simulink model "FK_IK"  (R2022b)
settings: Solver=FixedStepAuto  StartTime=0.0  StopTime=10.0  FixedStep=0.01  RelTol=1e-3
settings Model: Creator=Admin  LastModifiedBy=Admin

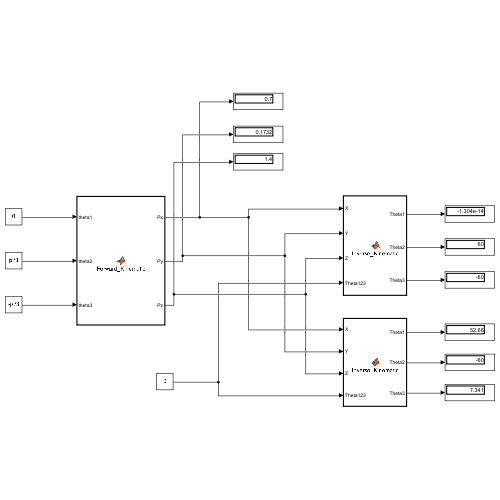
[thumbnail: Simulink's stored preview of the top-level diagram]
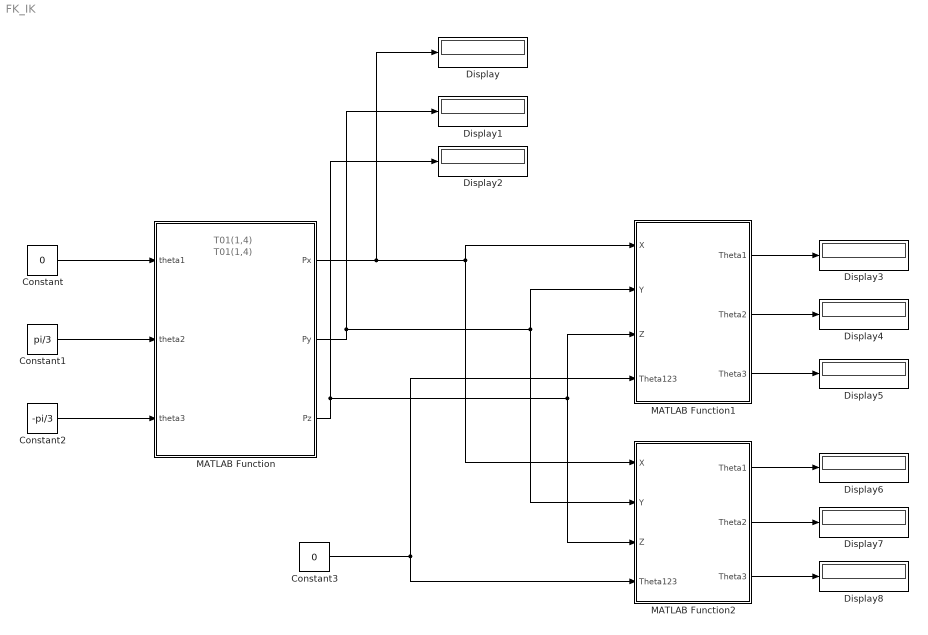
== system FK_IK ==
  note: T01(1,4)
  note: T01(1,4)
  Constant : Constant  Value=0
  Constant1 : Constant  Value=pi/3
  Constant2 : Constant  Value=-pi/3
  Constant3 : Constant  Value=0
  Display{,1..8} (9 alike) : Display
  MATLAB Function : MATLAB Function  TreatAsAtomicUnit=on
  MATLAB Function1 : MATLAB Function  TreatAsAtomicUnit=on
  MATLAB Function2 : MATLAB Function  TreatAsAtomicUnit=on
  wires:
  Constant/1 -> MATLAB Function/1(theta1)
  Constant1/1 -> MATLAB Function/2(theta2)
  Constant2/1 -> MATLAB Function/3(theta3)
  MATLAB Function/1(Px) -> MATLAB Function2/1(X), MATLAB Function1/1(X), Display/1
  MATLAB Function/2(Py) -> MATLAB Function2/2(Y), MATLAB Function1/2(Y), Display1/1
  MATLAB Function/3(Pz) -> MATLAB Function2/3(Z), MATLAB Function1/3(Z), Display2/1
  Constant3/1 -> MATLAB Function2/4(Theta123), MATLAB Function1/4(Theta123)
  MATLAB Function1/1(Theta1) -> Display3/1
  MATLAB Function1/2(Theta2) -> Display4/1
  MATLAB Function1/3(Theta3) -> Display5/1
  MATLAB Function2/3(Theta3) -> Display8/1
  MATLAB Function2/2(Theta2) -> Display7/1
  MATLAB Function2/1(Theta1) -> Display6/1

== matlab function FK_IK/MATLAB Function1 ==
  data: X input; Theta1 output; Y input; Z input; Theta123 input; Theta2 output; Theta3 output
function [Theta1,Theta2,Theta3] = Inverse_Kinematic(X,Y,Z, Theta123)
L0=0.2; L1=0.2; L2=0.25; L3=0.2; L4=0.15;
%% Tinh theta 2
N = X - L1 - L4*cosd(Theta123);
M = Y - L4*sind(Theta123);
C_T2 = (N^2 + M^2 - L2^2 - L3^2) / (2*L2*L3);
S_T2 = sqrt(abs(1 - C_T2^2));
Theta2 = atan2d(S_T2,C_T2);

%% Tinh theta 1
C_T1 = (N*(L2+L3*cosd(Theta2)) + M*L3*sind(Theta2)) / (L2^2+2*L2*L3*cosd(Theta2)+L3^2);
S_T1 = (M*(L2+L3*cosd(Theta2)) - N*L3*sind(Theta2)) / (L2^2+2*L2*L3*cosd(Theta2)+L3^2);
Theta1 = atan2d(S_T1,C_T1);

%% Tinh theta 3
Theta3 = Theta123 - Theta1 - Theta2;

== matlab function FK_IK/MATLAB Function ==
  data: theta1 input; Px output; theta2 input; theta3 input; Py output; Pz output
function [Px,Py,Pz] = Forward_Kinematic(theta1,theta2,theta3)
d1 = 0.3; d2 = 0.3; d3 = 0.3; d4 = 0.3;
L0=0.2; L1=0.2; L2=0.25; L3=0.2; L4=0.15;

%% The individual transformation:
%Ma tran chuyen doi tu he 0 sang 1
T01 = [cos(theta1), -sin(theta1), 0, L1;
       sin(theta1),  cos(theta1), 0,  0;
                  0,             0, 1, L0 + d1 + d2;
                  0,             0, 0,  1];
%Ma tran chuyen doi tu he 1 sang 2
T12 = [cos(theta2), -sin(theta2), 0, L2;
       sin(theta2),  cos(theta2), 0,  0;
                  0,             0, 1,  d3;
                  0,             0, 0,  1];
%Ma tran chuyen doi tu he 2 sang 3
T23 = [cos(theta3), -sin(theta3), 0, L3;
       sin(theta3),  cos(theta3), 0,  0;
                  0,             0, 1,  d4;
                  0,             0, 0,  1];
%Ma tran chuyen doi tu he 2 sang 3
T34 = [1, 0, 0, L4
       0, 1, 0,  0
       0, 0, 1,  0
       0, 0, 0,  1];
% %% The transformation matrix between frame(0) and frame (3)
T04=T01*T12*T23*T34;
%% Position of end-effector
Px = T04(1,4);
Py = T04(2,4);
Pz = T04(3,4);

== matlab function FK_IK/MATLAB Function2 ==
  data: X input; Theta1 output; Y input; Theta2 output; Theta3 output; Z input; Theta123 input
function [Theta1,Theta2,Theta3] = Inverse_Kinematic(X,Y,Z,Theta123)
L0=0.2; L1=0.2; L2=0.25; L3=0.2; L4=0.15;
%% Tinh theta 2
N = X - L1 - L4*cosd(Theta123);
M = Y - L4*sind(Theta123);
C_T2 = (N^2 + M^2 - L2^2 - L3^2) / (2*L2*L3);
S_T2 = -sqrt(abs(1 - C_T2^2));
Theta2 = atan2d(S_T2,C_T2);

%% Tinh theta 1
C_T1 = (N*(L2+L3*cosd(Theta2)) + M*L3*sind(Theta2)) / (L2^2+2*L2*L3*cosd(Theta2)+L3^2);
S_T1 = (M*(L2+L3*cosd(Theta2)) - N*L3*sind(Theta2)) / (L2^2+2*L2*L3*cosd(Theta2)+L3^2);
Theta1 = atan2d(S_T1,C_T1);

%% Tinh theta 3
Theta3 = Theta123 - Theta1 - Theta2;
